simulink model "gm_uz_pmsm_model_6LUT_pd_vnl"  (R2023b)
settings: Solver=FixedStepAuto  StartTime=0.0  StopTime=0.05  RelTol=1e-3
PreLoadFcn:
  | uz_pmsm_model_init_parameter
PostLoadFcn:
  | % Import the data from Excel for a lookup table
  | FluxMapData = readtable('C:\Users\Philipp\ultrazohm\ultrazohm_sw\ip_cores\uz_pmsm_model\FluxMapData_2023-05-26_13-07-57.csv');
  | % Row indices for lookup table
  | d_current_in_d_axis = FluxMapData(8:27,1:end);
  | % Column indices for lookup table
  | q_current_in_d_axis = FluxMapData(29:48,1:end);
  | % Output values for lookup table
  | d_Flux_d_axis = FluxMapData(50:69,1:end);
undefined symbols (not defined in the file or in its folder): ad1, ad2, ad3, ad4, ad5, ad6, aq1, aq2, aq3, aq4, aq5, aq6, d_current_d_Flux, d_current_q_Flux, entkopplung_dynamic, entkopplung_linear, entkopplung_static, Fid1_Giq1, Fid2_Giq2, Flux_d, Flux_q, friction_coefficient, inertia, Ki_Bo_d, Ki_Bo_q, Kp_Bo_d, Kp_Bo_q, L_d, L_q, Ldq, parameter_nachfuerung, polepair, praediktion_entkopplung_nonlinear, psi_pm, q_current_d_Flux, q_current_q_Flux, R_1, simulate_mechanical, simulate_nonlinear_modell, simulate_open_loop, static_friction_torque, tau_sum, ts, ts_regler
libraries: hdlmdlgenlib x21, simulink x2, slpidlib x2
(part 4 of 4)

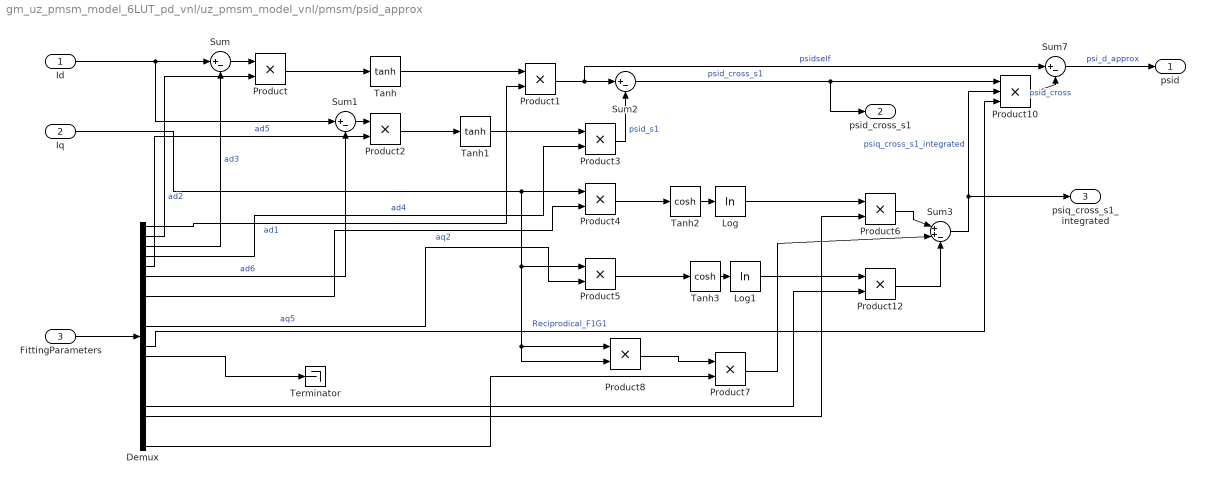
== system gm_uz_pmsm_model_6LUT_pd_vnl/uz_pmsm_model_vnl/pmsm/psid_approx ==
  Id : Inport
  Iq : Inport  Port=2
  FittingParameters : Inport  Port=3
  Demux : Demux  Outputs=23
  Log : Math  Operator=log  SignedPower=on
  Log1 : Math  Operator=log  SignedPower=on
  Product{,2,4..5,8} (5 alike) : Product  OutDataTypeStr=Inherit: Same as first input
  Product{1,3,6..7,12} (5 alike) : Product
  Product10 : Product  Inputs=3
  Sum{,1..2,7} (4 alike) : Sum  Inputs=|+-
  Sum3 : Sum  Inputs=|++-
  Tanh : Trigonometry  Operator=tanh
  Tanh1 : Trigonometry  Operator=tanh
  Tanh2 : Trigonometry  Operator=cosh
  Tanh3 : Trigonometry  Operator=cosh
  Terminator : Terminator
  psid : Outport
  psid_cross_s1 : Outport  Port=2
  psiq_cross_s1_integrated : Outport  Port=3
  wires:
  Demux/23 -> Product7/2
  Product5/1 -> Tanh3/1
  Product4/1 -> Tanh2/1
  Product2/1 -> Tanh1/1
  Product/1 -> Tanh/1
  Tanh1/1 -> Product3/1
  Tanh/1 -> Product1/1
  Log1/1 -> Product12/1
  Log/1 -> Product6/1
  Demux/13 -> Product10/3  "Reciprodical_F1G1"
  Demux/14 -> Terminator/1
  Sum7/1 -> psid/1  "psi_d_approx"
  Product10/1 -> Sum7/2  "psid_cross"
  Demux/8 -> Product4/2  "aq2"
  Demux/11 -> Product5/2  "aq5"
  Sum3/1 -> psiq_cross_s1_integrated/1, Product10/2  "psiq_cross_s1_integrated"
  Product12/1 -> Sum3/3
  Demux/19 -> Product12/2
  Product6/1 -> Sum3/1
  Demux/20 -> Product6/2
  Product7/1 -> Sum3/2
  Product8/1 -> Product7/1
  Tanh3/1 -> Log1/1
  Tanh2/1 -> Log/1
  Sum2/1 -> Product10/1, psid_cross_s1/1  "psid_cross_s1"
  Iq/1 -> Product4/1, Product5/1, Product8/1, Product8/2
  Product3/1 -> Sum2/2  "psid_s1"
  Id/1 -> Sum/1, Sum1/1
  Demux/6 -> Sum1/2  "ad6"
  Demux/5 -> Product2/2  "ad5"
  Sum1/1 -> Product2/1
  Demux/4 -> Product3/2  "ad4"
  Product1/1 -> Sum2/1, Sum7/1  "psidself"
  Demux/2 -> Product/2  "ad2"
  Sum/1 -> Product/1
  Demux/3 -> Sum/2  "ad3"
  Demux/1 -> Product1/2  "ad1"
  FittingParameters/1 -> Demux/1

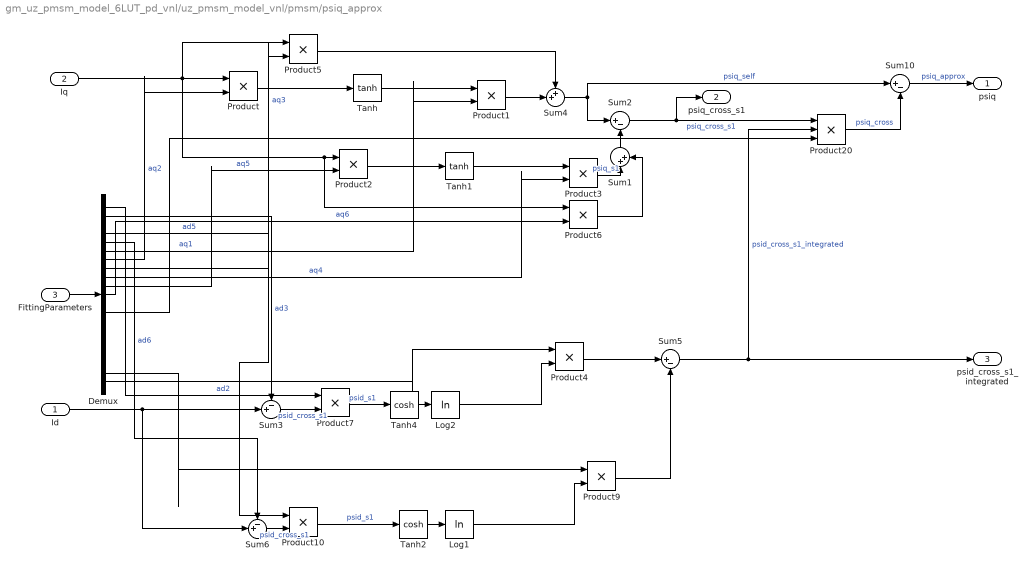
== system gm_uz_pmsm_model_6LUT_pd_vnl/uz_pmsm_model_vnl/pmsm/psiq_approx ==
  Id : Inport
  Iq : Inport  Port=2
  FittingParameters : Inport  Port=3
  Demux : Demux  Outputs=23
  Log1 : Math  Operator=log  SignedPower=on
  Log2 : Math  Operator=log  SignedPower=on
  Product{,2,7,10} (4 alike) : Product  OutDataTypeStr=Inherit: Same as first input
  Product{1,3..6,9} (6 alike) : Product
  Product20 : Product  Inputs=3
  Sum1 : Sum  Inputs=|++
  Sum10 : Sum  Inputs=|+-
  Sum2 : Sum  Inputs=|+-
  Sum3 : Sum  Inputs=-+|
  Sum4 : Sum  Inputs=++|
  Sum5 : Sum  Inputs=|+-
  Sum6 : Sum  Inputs=-+|
  Tanh : Trigonometry  Operator=tanh
  Tanh1 : Trigonometry  Operator=tanh
  Tanh2 : Trigonometry  Operator=cosh
  Tanh4 : Trigonometry  Operator=cosh
  psiq : Outport
  psiq_cross_s1 : Outport  Port=2
  psid_cross_s1_integrated : Outport  Port=3
  wires:
  Product/1 -> Tanh/1
  Product2/1 -> Tanh1/1
  Tanh/1 -> Product1/1
  Tanh1/1 -> Product3/1
  Log2/1 -> Product4/2
  Log1/1 -> Product9/2
  Demux/14 -> Product20/3
  Sum10/1 -> psiq/1  "psiq_approx"
  Product20/1 -> Sum10/2  "psiq_cross"
  Sum5/1 -> Product20/2, psid_cross_s1_integrated/1  "psid_cross_s1_integrated"
  Id/1 -> Sum3/2, Sum6/2
  Demux/6 -> Sum6/1  "ad6"
  Demux/5 -> Product10/1  "ad5"
  Demux/2 -> Product7/1  "ad2"
  Demux/3 -> Sum3/1  "ad3"
  Sum6/1 -> Product10/2  "psid_cross_s1"
  Demux/21 -> Product9/1
  Tanh2/1 -> Log1/1
  Product10/1 -> Tanh2/1  "psid_s1"
  Product9/1 -> Sum5/2
  Product4/1 -> Sum5/1
  Product7/1 -> Tanh4/1  "psid_s1"
  Sum3/1 -> Product7/2  "psid_cross_s1"
  Product6/1 -> Sum1/2
  Product3/1 -> Sum1/1  "psiq_s1"
  Sum1/1 -> Sum2/2
  Sum4/1 -> Sum2/1, Sum10/1  "psiq_self"
  Product5/1 -> Sum4/1
  Product1/1 -> Sum4/2
  Demux/22 -> Product4/1
  Tanh4/1 -> Log2/1
  Demux/9 -> Product5/2  "aq3"
  Iq/1 -> Product5/1, Product/1, Product6/1, Product2/1
  Demux/7 -> Product1/2  "aq1"
  Demux/11 -> Product2/2  "aq5"
  Demux/8 -> Product/2  "aq2"
  Demux/12 -> Product6/2  "aq6"
  Demux/10 -> Product3/2  "aq4"
  Sum2/1 -> psiq_cross_s1/1, Product20/1  "psiq_cross_s1"
  FittingParameters/1 -> Demux/1

== matlab function gm_uz_pmsm_model_6LUT_pd_vnl/Compare/Assert_outputs/RelErrCheck/RelativeErrorCheck  ==
  data: P input; y output; R input; ToleranceValue parameter double
% Check if the relative error of R with respect to P is below
% ToleranceValue
% P, R are floating-point
function y = relErrCheck(P,R, ToleranceValue)
    tol = ToleranceValue;
    sz = numel(P);
    assert(sz == numel(R), 'Inputs P and R have different sizes.');
    y = false(1, sz);

    for ii=1:sz
        if (isnan(P(ii)) || isnan(R(ii)))
            if (isnan(P(ii)) && isnan(R(ii)))
                y(ii) = true;
            end
        elseif (isinf(P(ii)) || isinf(R(ii)))
            y(ii) = (P(ii) == R(ii));
        elseif (P(ii) == 0)
            y(ii) = (R(ii) == 0);
        else
            absdiff = abs(P(ii) - R(ii));
            relerr = absdiff/abs(P(ii));
            y(ii) = (relerr <= tol);
        end
    end
end
